simulink model "SPWm"  (R2022a)
settings: Solver=VariableStepAuto  StartTime=0.0  StopTime=10.0  RelTol=1e-3
libraries: spsControlledVoltageSourceLib x2, simulink x2, spsAsynchronousMachineSIUnitsLib x1, spsGroundLib x1, spsThreePhaseVIMeasurementLib x1, spspowerguiLib x1
settings Model: Creator=Kemalettin  LastModifiedBy=Kemalettin

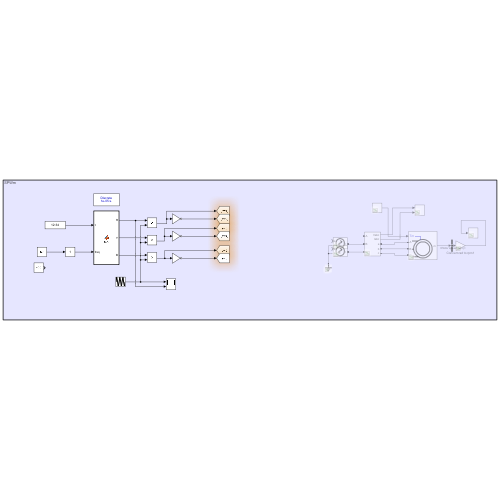
[thumbnail: Simulink's stored preview of the top-level diagram]
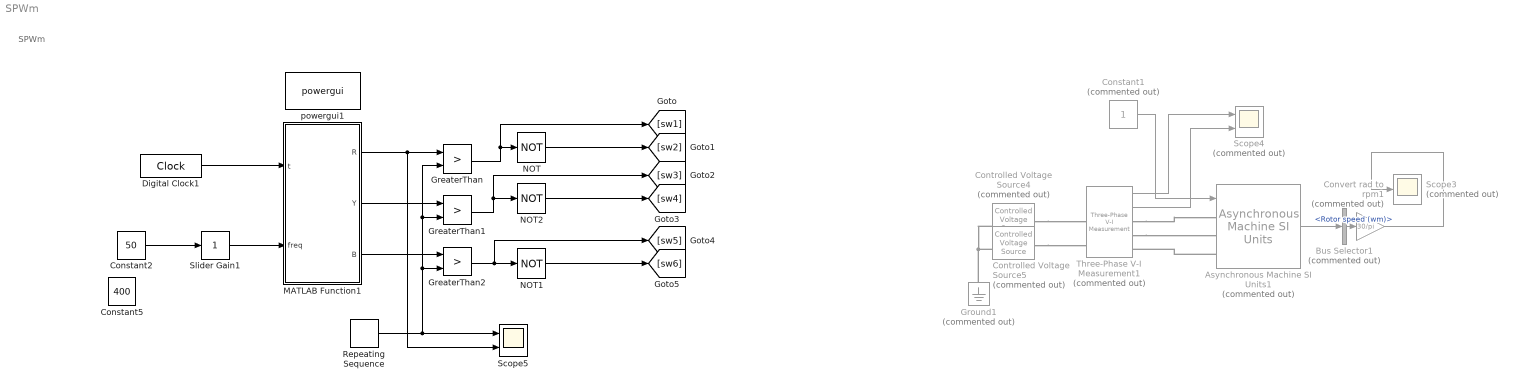
== system SPWm ==
  note: SPWm
  Asynchronous Machine SI Units1 : spsAsynchronousMachineSIUnitsLib/Asynchronous Machine SI Units  Commented=on  RotorType=Squirrel-cage  PresetModel="16:  10 HP (7.5KW)  400 V 50Hz 1440 RPM"  MechanicalLoad=Torque Tm  ShowDetailedParameters=on  ReferenceFrame=Rotor  Units=SI  MeasurementBus=off  NominalParameters=[7500 400 50]  VoltageRatio=1  Stator=[0.7384 0.003045]  Rotor=[0.7402 0.003045]  Cage1=[0.4155 0.002066]  Cage2=[0.4168 0.0003495]  Lm=0.1241  Mechanical=[0.0343 0.000503 2]  PolePairs=2  InitialConditions=[0 0 0 0 0 0 0 0]  SimulateSaturation=off  Saturation=[14.03593122, 27.81365428, 53.79336849, 72.68890987, 97.98006896, 148.6815601, 215.7428561, 302.9841135, 428.7778367 ; 230, 322, 414, 460, 506, 552, 598, 644, 690]  LoadFlowParameters=1492000  TsPowergui=0  TsBlock=-1  IterativeModel=Trapezoidal non iterative  IterativeDiscreteModel=Trapezoidal non iterative  Pmec=1.492e+006
  Bus Selector1 : BusSelector  Commented=on  OutputSignals=Mechanical.Rotor speed (wm)
  Constant1 : Constant  Commented=on
  Constant2 : Constant  Value=50
  Constant5 : Constant  Value=400
  Controlled Voltage Source4 : spsControlledVoltageSourceLib/Controlled Voltage Source  Commented=on  Initialize=on  Source_Type=AC  Amplitude=0  Phase=0  Frequency=0  Measurements=None
  Controlled Voltage Source5 : spsControlledVoltageSourceLib/Controlled Voltage Source  Commented=on  Initialize=on  Source_Type=AC  Amplitude=0  Phase=0  Frequency=0  Measurements=None
  Convert rad to rpm1 : Gain  Commented=on  Gain=30/pi
  Digital Clock1 : DigitalClock  SampleTime=1e-5
  GreaterThan : RelationalOperator  Operator=>  OutDataTypeStr=boolean  RndMeth=Simplest  InputSameDT=off
  GreaterThan1 : RelationalOperator  Operator=>  OutDataTypeStr=boolean  RndMeth=Simplest  InputSameDT=off
  GreaterThan2 : RelationalOperator  Operator=>  OutDataTypeStr=boolean  RndMeth=Simplest  InputSameDT=off
  Ground1 : spsGroundLib/Ground  Commented=on  LConnTagsString=a
  MATLAB Function1 : MATLAB Function  TreatAsAtomicUnit=on
  NOT : Logic  Operator=NOT  IconShape=distinctive  AllPortsSameDT=off  OutDataTypeStr=boolean
  NOT1 : Logic  Operator=NOT  IconShape=distinctive  AllPortsSameDT=off  OutDataTypeStr=boolean
  NOT2 : Logic  Operator=NOT  IconShape=distinctive  AllPortsSameDT=off  OutDataTypeStr=boolean
  Repeating Sequence : simulink/Sources/Repeating Sequence  rep_seq_t=[0 .25 .50 .75 1]*1/5000  rep_seq_y=[0 1 0 -1 0]
  Scope3 : Scope  Commented=on
  Scope4 : Scope  Commented=on  NumInputPorts=2
  Scope5 : Scope  NumInputPorts=2
  Slider Gain1 : simulink/Math Operations/Slider Gain  gain=1  low=0  high=1
  Three-Phase V-I Measurement1 : spsThreePhaseVIMeasurementLib/Three-Phase V-I Measurement  Commented=on  VoltageMeasurement=phase-to-ground  SetLabelV=off  LabelV=Vabc  Vpu=off  VpuLL=off  CurrentMeasurement=yes  SetLabelI=off  LabelI=Iabc  Ipu=off  Pbase=100e6  Vbase=500e3  OutputType=Complex  PhasorSimulation=off  PSBequivalent=0
  powergui1 : spspowerguiLib/powergui  Priority=1  SimulationMode=Discrete  SampleTime=1e-5  frequency=60  Iterations=50  frequencyindice=50  Pbase=100e6  ErrMax=1e-4  UnitsV=kV  UnitsW=MW  buscounter=0  FunctionMessages=off  echomessages=off  EnableUseOfTLC=off  CurrentSourceSwitches=off  DisableSnubberDevices=off  DisableRonSwitches=off  DisableVfSwitches=off  DisplayEquations=off  AutomaticDiscreteSolvers=off  SolverType=Tustin/Backward Euler (TBE)  Interpol=off  ExternalGateDelay=off  methode=off  Ts=100  x0status=blocks  SPID=on  SwTol=0  HookPort=off  NonlinearTolerance=1e-4  nMaxIteration=100  ContinueOnMaxIteration=off  RestoreLinks=warning  ResistiveCurrentMeasurement=off  Frange=[0:2:500]  Ylog=off  Xlog=on  ShowGrid=off  save=off  variable=ZData  structure=0  ZoomFFT=off  StartTime=0.0  cycles=1  DisplayStyle=1  fundamental=60  FreqAxis=off  MaxFrequency=1000  frequencyindicesteady=1  RmsSteady=1  display=off
  wires:
  Constant2/1 -> Slider Gain1/1
  MATLAB Function1/1(R) -> Scope5/2, GreaterThan/1
  GreaterThan/1 -> [sw1], NOT/1
  MATLAB Function1/3(B) -> GreaterThan2/1
  NOT2/1 -> [sw4]
  GreaterThan2/1 -> [sw5], NOT1/1
  MATLAB Function1/2(Y) -> GreaterThan1/1
  NOT1/1 -> [sw6]
  Repeating Sequence/1 -> Scope5/1, GreaterThan/2, GreaterThan1/2, GreaterThan2/2
  Digital Clock1/1 -> MATLAB Function1/1(t)
  Slider Gain1/1 -> MATLAB Function1/2(freq)
  Bus Selector1/1 -> Convert rad to rpm1/1  "<Rotor speed (wm)>"
  GreaterThan1/1 -> [sw3], NOT2/1
  NOT/1 -> [sw2]
  Convert rad to rpm1/1 -> Scope3/1
  Three-Phase V-I Measurement1/1 -> Scope4/1
  Three-Phase V-I Measurement1/2 -> Scope4/2
  Asynchronous Machine SI Units1/1 -> Bus Selector1/1
  Constant1/1 -> Asynchronous Machine SI Units1/1
  connections:
  Controlled Voltage Source5/LConn1 -- Controlled Voltage Source4/LConn1 -- Ground1/LConn1
  Three-Phase V-I Measurement1/RConn1 -- Asynchronous Machine SI Units1/LConn1
  Controlled Voltage Source4/RConn1 -- Three-Phase V-I Measurement1/LConn2
  Controlled Voltage Source5/RConn1 -- Three-Phase V-I Measurement1/LConn3
  Three-Phase V-I Measurement1/RConn2 -- Asynchronous Machine SI Units1/LConn2
  Asynchronous Machine SI Units1/LConn3 -- Three-Phase V-I Measurement1/RConn3

== matlab function SPWm/MATLAB Function1 ==
  data: t input; R output; freq input; Y output; B output
function [R,Y,B] = fcn(t,freq)
omega = 2 * pi *freq;
R = sin(omega * t) * freq/60;
Y = sin(omega * t+120*pi/180) * freq/60;
B = sin(omega * t+240*pi/180) * freq/60;
